simulink model "Steuerung"  (R2018a)
settings: Solver=ode1  StartTime=0.0  StopTime=inf  FixedStep=1/10  RelTol=1e-3  EnableMultiTasking=on
undefined symbols (not defined in the file): gray
libraries: PiCar_library x3, simulink x3
settings Model: SimulationMode=external  Creator=raspberry  LastModifiedBy=Herib
settings SolverCC: PositivePriorityOrder=on
settings OptimizationCC: PassReuseOutputArgsAs=Individual arguments  MaxStackSize=64
settings DebuggingCC: ParameterTunabilityLossMsg=error
settings HardwareCC: ProdBitPerPointer=32  ProdBitPerSizeT=32  ProdBitPerPtrDiffT=32  ProdLargestAtomicInteger=Long  ProdLargestAtomicFloat=Double  ProdWordSize=32  ProdHWDeviceType=ARM Compatible->ARM Cortex
settings SFSimCC: MATLABDynamicMemAlloc=off
settings RTWCC: SystemTargetFile=ert.tlc  HardwareBoard=Raspberry Pi  TLCOptions="-aInlineSetEventsForThisBaseRateFcn=TLC_FALSE -aSuppressMultiTaskScheduler=TLC_FALSE  -aRateBasedStepFcn=0"  TemplateMakefile=ert_default_tmf  Toolchain=GNU GCC Raspberry Pi
settings RTWCC: CustomTerminator=|
  | /* Send ALL_LED_OFF Signal to all PWM driver chip address
  | See PCA9685 user manual, section 7.3.4
  | Set Chip in sleep mode, section 7.3.1
  | Reset the PWM ON/OFF states for all LEDs */
  | 
  | int fd;
  | 
  | fd = wiringPiI2CSetup(0x70);
  | wiringPiI2CWriteReg8(fd, 0x00, 0x11); // sleep mode
  | wiringPiI2CWriteReg8(fd, 0xFD, 0x10); // all LED off
  | wiringPiI2CWriteReg8(fd, 0xFC, 0x00);
  | wiringPiI2CWriteReg8(fd, 0xFB, 0x00);
  | wiringPiI2CWriteReg8(fd, 0xFA, 0x00);
settings CodeAppCC: ForceParamTrailComments=on  IgnoreCustomStorageClasses=off  OperatorAnnotations=on  SimulinkDataObjDesc=on  SFDataObjDesc=on  MATLABFcnDesc=on  InsertBlockDesc=on  StateflowObjectComments=on  MATLABSourceComments=on
settings ERTTargetCC: SupportVariableSizeSignals=on

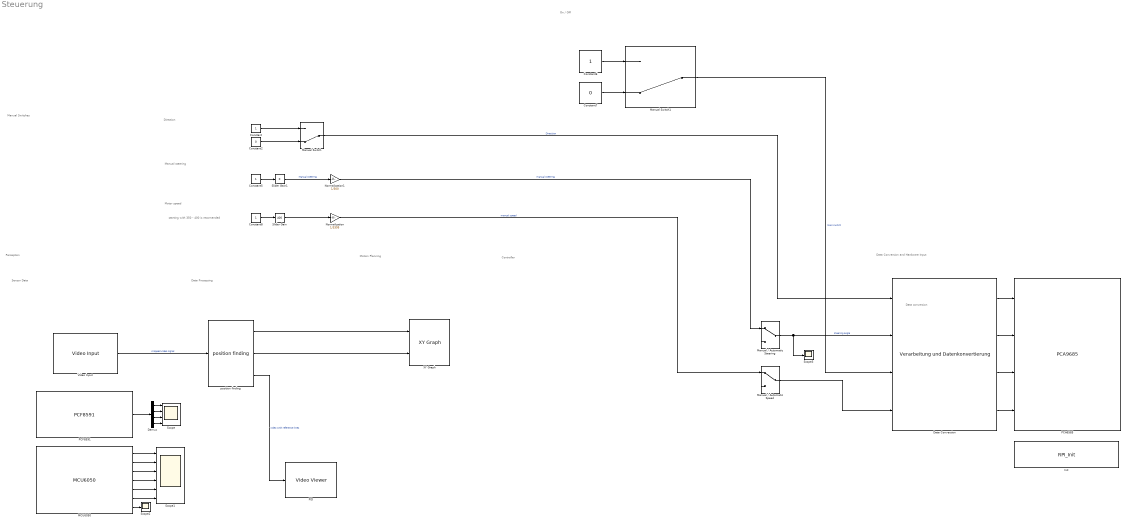
== system Steuerung ==
  note: starting with 350 - 400 is recomended
  note: Data Conversion and Hardware Input
  note: Data conversion
  note: Manual Switches
  note: Motion Planning
  note: Perception
  note: Controller
  note: Data Processing
  note: Sensor Data
  note: Manual steering
  note: Motor speed
  note: Direction
  note: On / Off
  Constant{,5..6,8} (4 alike) : Constant
  Constant2 : Constant  Value=0
  Constant7 : Constant  Value=0
  Data Conversion : PiCar_library/Verarbeitung und Datenkonvertierung
  Demux : Demux
  Init : S-Function  Priority=1  InitFcn=try, set_param(gcb,'FunctionName','RPI_Init'), end  FunctionName=RPI_Init  SFunctionModules=RPI_Init_wrapper  SFunctionDeploymentMode=off  EnableBusSupport=off  mask(S-Function Builder){}
      mask help: Simulink:masks:SFunctionBuilder_MD
      mask init:
      | val = [[.9  0.75 0.75 1 1 .9 .9 1]',[1 1 0.75 0.75 .9 .9 1 .9]'];try , sys = get_param(gcb,'SfunBuilderFcnName');if isempty(sys), sys = get_param(gcb,'FunctionName'); end,catch, sys = get_param(gcb,'FunctionName'); end
      settings: CopyFcn=set_param(gcbh,'LinkStatus','none')  PreSaveFcn=try, set_param(gcb,'FunctionName','RPI_Init'), end  OpenFcn=sfunctionwizard(gcbh)
      mask Display:
      | plot(val(:,1),val(:,2))
      | disp(sys)
  MCU6050 : S-Function  InitFcn=try, set_param(gcb,'FunctionName','MCU6050'), end  FunctionName=MCU6050  SFunctionModules=MCU6050_wrapper  SFunctionDeploymentMode=off  EnableBusSupport=off  mask(S-Function Builder){}
      mask help: Simulink:masks:SFunctionBuilder_MD
      mask init: same as Steuerung/Init
      settings: CopyFcn=set_param(gcbh,'LinkStatus','none')  PreSaveFcn=try, set_param(gcb,'FunctionName','MCU6050'), end  OpenFcn=sfunctionwizard(gcbh)
      mask Display: plot(val(:,1),val(:,2)),disp(sys), port_label('output',1,'ax'), port_label('output',2,'ay'), port_label('output',3,'az'), port_label('output',4,'omx'), port_label('output',5,'omy'), port_label('output',6,'omz'), port_label('output',7,'temp')
  Manual / Automatic Speed : ManualSwitch
  Manual / Automatic Steering : ManualSwitch
  Manual Switch : ManualSwitch  CurrentSetting=0
  Manual Switch1 : ManualSwitch  CurrentSetting=0
  Normalization : Gain  Gain=1/3395
  Normalization1 : Gain  Gain=1/300
  PCA6585 : S-Function  InitFcn=try, set_param(gcb,'FunctionName','PCA9685'), end  FunctionName=PCA9685  SFunctionModules=PCA9685_wrapper  SFunctionDeploymentMode=off  EnableBusSupport=off  mask(S-Function Builder){}
      mask help: Simulink:masks:SFunctionBuilder_MD
      mask init: same as Steuerung/Init
      settings: CopyFcn=set_param(gcbh,'LinkStatus','none')  PreSaveFcn=try, set_param(gcb,'FunctionName','PCA9685'), end  OpenFcn=sfunctionwizard(gcbh)
      mask Display: plot(val(:,1),val(:,2)),disp(sys), port_label('input',1,'IN_1'), port_label('input',2,'IN_2'), port_label('input',3,'PWM'), port_label('input',4,'SERVO')
  PCF8591 : S-Function  InitFcn=try, set_param(gcb,'FunctionName','PCF8591'), end  FunctionName=PCF8591  SFunctionModules=PCF8591_wrapper  SFunctionDeploymentMode=off  EnableBusSupport=off  mask(S-Function Builder){}
      mask help: Simulink:masks:SFunctionBuilder_MD
      mask init: same as Steuerung/Init
      settings: CopyFcn=set_param(gcbh,'LinkStatus','none')  PreSaveFcn=try, set_param(gcb,'FunctionName','PCF8591'), end  OpenFcn=sfunctionwizard(gcbh)
      mask Display: plot(val(:,1),val(:,2)),disp(sys), port_label('output',1,'PCF8591_out')
  PID : VideoViewer  colormapValue=gray(256)  FigPos=[1325 441 555 306]
  Scope : Scope  NumInputPorts=4
  Scope1 : Scope  NumInputPorts=6
  Scope2 : Scope
  Scope3 : Scope
  Slider Gain : simulink/Math Operations/Slider Gain  gain=400  low=0  high=3395
  Slider Gain1 : simulink/Math Operations/Slider Gain  gain=0  low=-300  high=300
  Video Input : PiCar_library/Video Input
  XY Graph : simulink/Sinks/XY Graph  xmin=0  xmax=1  ymin=-0.5  ymax=0.5  st=1/10
  position finding : PiCar_library/position finding
      link override BW thresh: Value=0.6695652173913
      link override auto thresh: Value=1
  wires:
  Constant/1 -> Manual Switch/1
  Constant2/1 -> Manual Switch/2
  Constant7/1 -> Manual Switch1/2
  Constant6/1 -> Manual Switch1/1
  Constant8/1 -> Slider Gain/1
  Slider Gain1/1 -> Normalization1/1  "Manual steering"
  Constant5/1 -> Slider Gain1/1
  Demux/3 -> Scope/3
  Demux/4 -> Scope/4
  PCF8591/1 -> Demux/1
  MCU6050/2 -> Scope1/2
  MCU6050/3 -> Scope1/3
  MCU6050/1 -> Scope1/1
  MCU6050/4 -> Scope1/4
  MCU6050/5 -> Scope1/5
  MCU6050/6 -> Scope1/6
  MCU6050/7 -> Scope2/1
  Manual Switch/1 -> Data Conversion/1  "Direction"
  Manual / Automatic Steering/1 -> Data Conversion/2, Scope3/1  "steering angle"
  Manual Switch1/1 -> Data Conversion/3  "main switch"
  Data Conversion/1 -> PCA6585/1
  Data Conversion/2 -> PCA6585/2
  Data Conversion/3 -> PCA6585/3
  Data Conversion/4 -> PCA6585/4
  Video Input/1 -> position finding/1  "cropped video signal"
  ? -> Manual / Automatic Steering/2  "steering angle"
  Slider Gain/1 -> Normalization/1
  position finding/3 -> PID/1  "video with reference lines"
  Normalization/1 -> Manual / Automatic Speed/1  "manual speed"
  Normalization1/1 -> Manual / Automatic Steering/1  "manual steering"
  Demux/1 -> Scope/1
  Demux/2 -> Scope/2
  Manual / Automatic Speed/1 -> Data Conversion/4
  ? -> Manual / Automatic Speed/2
  position finding/1 -> XY Graph/1
  position finding/2 -> XY Graph/2
